simulink subsystem "Process_Coordinates"  (R2022b)
settings: Solver=VariableStepAuto  StartTime=0.0  StopTime=10.0  RelTol=1e-3
settings Model: Creator=User  LastModifiedBy=User

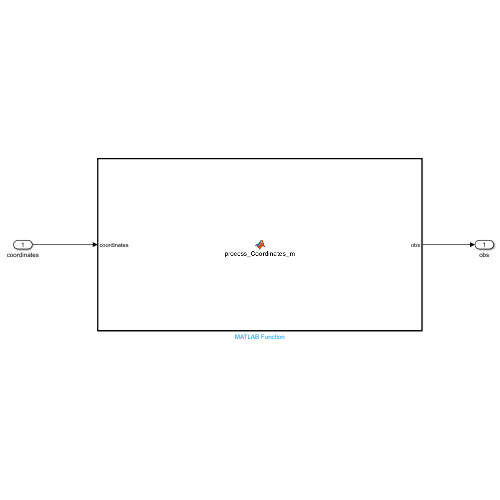
[thumbnail: Simulink's stored preview of the top-level diagram]
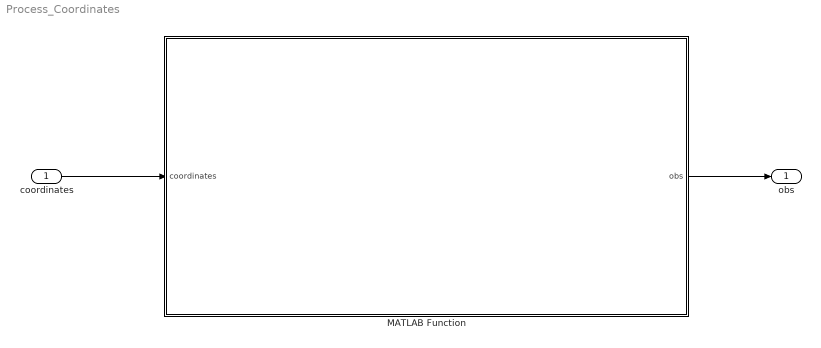
== system Process_Coordinates ==
  coordinates : Inport
  MATLAB Function : MATLAB Function  TreatAsAtomicUnit=on
  obs : Outport
  wires:
  coordinates/1 -> MATLAB Function/1(coordinates)
  MATLAB Function/1(obs) -> obs/1

== matlab function Process_Coordinates/MATLAB Function ==
  data: coordinates input; obs output
function obs = process_Coordinates_m(coordinates)
    obs = process_Coordinates(coordinates);
    
end
